simulink model "NIVEL_2_COMPLETO"  (R2024b)
settings: Solver=VariableStepAuto  StartTime=0.0  StopTime=10.0  RelTol=1e-3
settings Model: Creator=juani  LastModifiedBy=juani

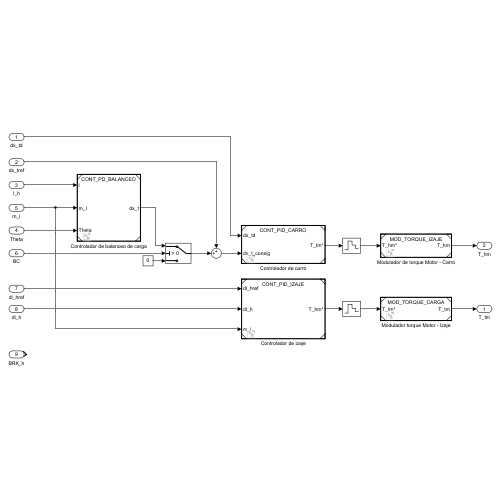
[thumbnail: Simulink's stored preview of the top-level diagram]
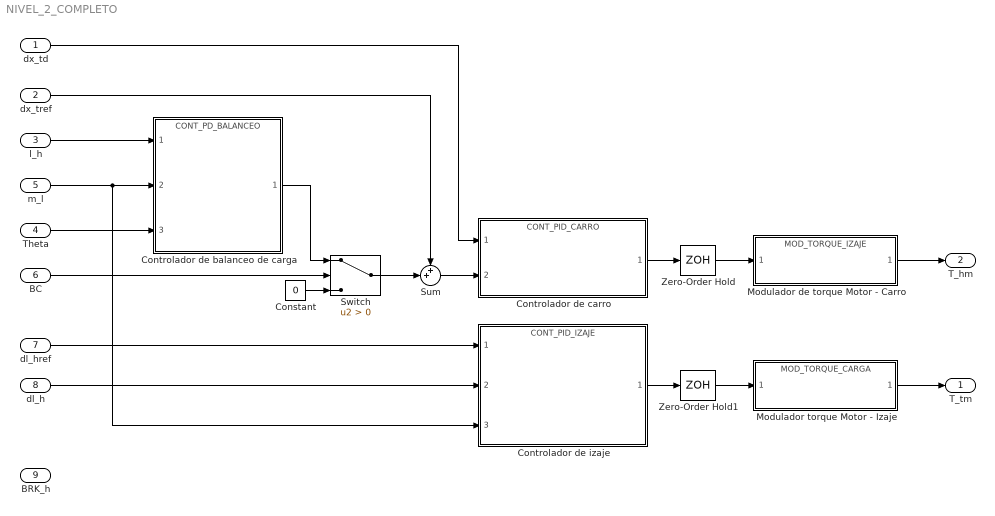
== system NIVEL_2_COMPLETO ==
  dx_td : Inport
  dx_tref : Inport  Port=2
  l_h : Inport  Port=3
  Theta : Inport  Port=4
  m_l : Inport  Port=5
  BC : Inport  Port=6
  dl_href : Inport  Port=7
  dl_h : Inport  Port=8
  BRK_h : Inport  Port=9
  Constant : Constant  Value=0
  Controlador de balanceo de carga : ModelReference  ModelNameDialog=CONT_PD_BALANCEO.slx  SimulationMode=Normal  ModelReferenceVersion=1.8
  Controlador de carro : ModelReference  ModelNameDialog=CONT_PID_CARRO.slx  SimulationMode=Normal  ModelReferenceVersion=1.5
  Controlador de izaje : ModelReference  ModelNameDialog=CONT_PID_IZAJE.slx  SimulationMode=Normal  ModelReferenceVersion=1.7
  Modulador de torque Motor - Carro : ModelReference  ModelNameDialog=MOD_TORQUE_IZAJE.slx  SimulationMode=Normal  ModelReferenceVersion=1.2
  Modulador torque Motor - Izaje : ModelReference  ModelNameDialog=MOD_TORQUE_CARGA.slx  SimulationMode=Normal  ModelReferenceVersion=1.2
  Sum : Sum  Inputs=++|
  Switch : Switch  Criteria=u2 > Threshold  SaturateOnIntegerOverflow=off  InputSameDT=off
  Zero-Order Hold : ZeroOrderHold  SampleTime=-1
  Zero-Order Hold1 : ZeroOrderHold  SampleTime=-1
  T_tm : Outport
  T_hm : Outport  Port=2
  wires:
  dx_td/1 -> Controlador de carro/1
  l_h/1 -> Controlador de balanceo de carga/1
  m_l/1 -> Controlador de izaje/3, Controlador de balanceo de carga/2
  Theta/1 -> Controlador de balanceo de carga/3
  Controlador de balanceo de carga/1 -> Switch/1
  BC/1 -> Switch/2
  Constant/1 -> Switch/3
  Switch/1 -> Sum/2
  dx_tref/1 -> Sum/1
  Sum/1 -> Controlador de carro/2
  Controlador de carro/1 -> Zero-Order Hold/1
  Zero-Order Hold/1 -> Modulador de torque Motor - Carro/1
  Controlador de izaje/1 -> Zero-Order Hold1/1
  Zero-Order Hold1/1 -> Modulador torque Motor - Izaje/1
  dl_href/1 -> Controlador de izaje/1
  dl_h/1 -> Controlador de izaje/2
  Modulador de torque Motor - Carro/1 -> T_hm/1
  Modulador torque Motor - Izaje/1 -> T_tm/1
